simulink model "FM_RXTX_Audio_File"  (R2020b)
settings: Solver=VariableStepAuto  StartTime=0.0  StopTime=10  RelTol=1e-3
undefined symbols (not defined in the file or in its folder): designMultirateFIR
libraries: dspmlti4 x2, commanabbnd3 x2, dspvision x1, dspobslib x1
settings Model: Creator=Guillaume  LastModifiedBy=Guillaume

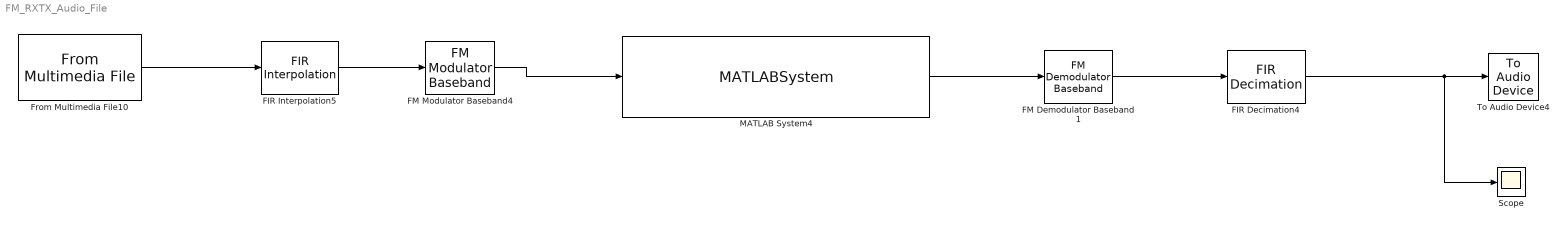
== system FM_RXTX_Audio_File ==
  FIR Decimation4 : dspmlti4/FIR Decimation  FilterSource=Auto  h=designMultirateFIR(1,2)  D=30  filtStruct=Direct form  FilterObject=FDECIM  InputProcessing=Columns as channels (frame based)  framing=Enforce single-rate processing  inputOffset=0  outputBufInitCond=0  roundingMode=Floor  overflowMode=off  firstCoeffDataTypeStr=Inherit: Same word length as input  firstCoeffMin=[]  firstCoeffMax=[]  firstCoeffLastDataTypeStr=Inherit: Same word length as input  outputDataTypeStr=Inherit: Same as accumulator  outputMin=[]  outputMax=[]  outputLastDataTypeStr=Inherit: Same as accumulator
  FIR Interpolation5 : dspmlti4/FIR Interpolation  FilterSource=Auto  PrivateCoeffs=0  h=designMultirateFIR(3,1)  L=30  FilterObject=FINTERP  InputProcessing=Columns as channels (frame based)  framing=Enforce single-rate processing  outputBufInitCond=0  roundingMode=Floor  overflowMode=off  firstCoeffDataTypeStr=Inherit: Same word length as input  firstCoeffMin=[]  firstCoeffMax=[]  firstCoeffLastDataTypeStr=Inherit: Same word length as input  outputDataTypeStr=Inherit: Same as accumulator  outputMin=[]  outputMax=[]  outputLastDataTypeStr=Inherit: Same as accumulator
  FM Demodulator Baseband 1 : commanabbnd3/FM Demodulator Baseband   FrequencyDeviation=75e3  SimulateUsing=Code generation
      settings: SourceProductBaseCode=CM
  FM Modulator Baseband4 : commanabbnd3/FM Modulator Baseband  FrequencyDeviation=75e3  SimulateUsing=Code generation
      settings: SourceProductBaseCode=CM
  From Multimedia File10 : dspvision/From Multimedia File  inputFilename=F:\Documents\MATLAB\LimeSDR\LimeSDR_Mini_Matlab_Github_2022\music1_mono48kHz.wav  readRange=[1 Inf]  loop=on  numPlays=inf  outputStreams=Audio only  videoDataType=single  audioDataType=double  inheritSampleTime=on  userDefinedSampleTime=1/30  noAudioOutput=off  isIntensityVideo=off  fourcc=RGB  colorVideoFormat=One multidimensional signal  outputEOF=off  dataOrg=Column-major  audioFrameSize=600  computeAudioFrameSize=off  outSamplingMode=Sample based
  MATLAB System4 : MATLABSystem  System=limeSDR_Simulink_Wrapper_2022  enable_rx0=on  rx0_antenna=3  rx0_bandwidth=1.5  rx0_gain=10  rx_frequency=868e6  rx_samplerate=1.44e6  rx_timeout_ms=5000  rx_step_size=18000  enable_tx0=on  tx0_antenna=2  tx0_bandwidth=1.5  tx0_gain=10  tx_frequency=868e6  tx_samplerate=1.44e6  tx_timeout_ms=5000  tx_step_size=18000
      mask Type: limeSDR_Simulink_Wrapper_2022
      mask Display:
      | disp('LimeSDR mini');
      | port_label('input',1,'TX0 Samples');
      | port_label('output',1,'RX0 Samples');
  Scope : Scope
  To Audio Device4 : dspobslib/To Audio Device  deviceName=Default  inheritSampleRate=on  sampleRate=44100  deviceDatatype=Determine from input data type  autoBufferSize=on  bufferSize=4096  queueDuration=1.0  defaultOutputChannelMapping=on  outputChannelMapping=1  outputNumUnderrunSamples=off
      settings: SourceProductBaseCode=DS
  wires:
  From Multimedia File10/1 -> FIR Interpolation5/1
  FIR Interpolation5/1 -> FM Modulator Baseband4/1
  FM Modulator Baseband4/1 -> MATLAB System4/1
  MATLAB System4/1 -> FM Demodulator Baseband 1/1
  FM Demodulator Baseband 1/1 -> FIR Decimation4/1
  FIR Decimation4/1 -> Scope/1, To Audio Device4/1
